simulink model "problem_6"  (R2020b)
settings: Solver=VariableStepAuto  StartTime=0.0  StopTime=30  RelTol=1e-3
PreLoadFcn:
  | Preload_values
settings Model: Creator=hp  LastModifiedBy=hp

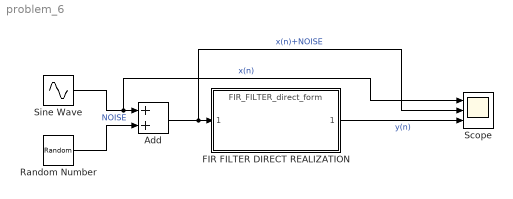
== system problem_6 ==
  Add : Sum
  FIR FILTER DIRECT REALIZATION : ModelReference  ModelNameDialog=FIR_FILTER_direct_form  SimulationMode=Normal  ModelReferenceVersion=1.10
  Random Number : RandomNumber  Variance=0.01  SampleTime=0.1
  Scope : Scope  NumInputPorts=3
  Sine Wave : Sin  SineType=Sample based  SampleTime=0.5
  wires:
  Add/1 -> Scope/2, FIR FILTER DIRECT REALIZATION/1  "x(n)+NOISE"
  Sine Wave/1 -> Scope/1, Add/1  "x(n)"
  Random Number/1 -> Add/2  "NOISE"
  FIR FILTER DIRECT REALIZATION/1 -> Scope/3  "y(n)"
